simulink subsystem "motorModel"  (R2026a)
settings: Solver=VariableStepAuto
settings Model: Creator=maxhu  LastModifiedBy=maxhu

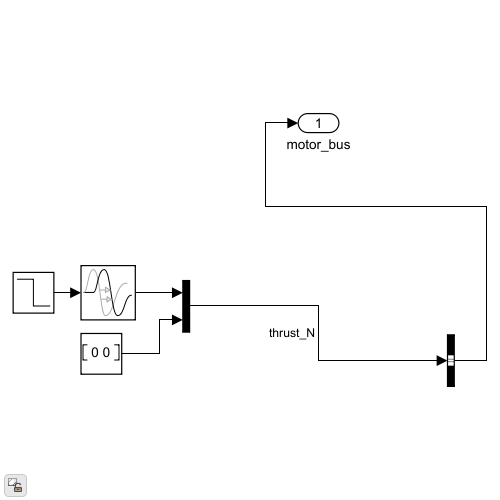
[thumbnail: Simulink's stored preview of the top-level diagram]
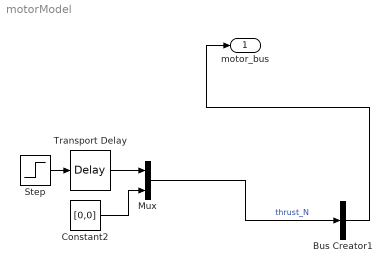
== system motorModel ==
  Bus Creator1 : BusCreator  Inputs=1
  Constant2 : Constant  Value=[0,0]
  Mux : Mux  Inputs=2
  Step : Step  Time=5  InitialValue=2000  FinalValue=0  SampleTime=0
  Transport Delay : TransportDelay  DelayTime=10
  motor_bus : Outport
  wires:
  Mux/1 -> Bus Creator1/1  "thrust_N"
  Constant2/1 -> Mux/2
  Transport Delay/1 -> Mux/1
  Step/1 -> Transport Delay/1
  Bus Creator1/1 -> motor_bus/1
